simulink model "sk_Depositos_control"  (Simulink 8.9)
settings: Solver=ode45  StartTime=0.0  StopTime=tsim  RelTol=1e-3  EnableMultiTasking=on
values from neighbouring files (symbols this model uses):
  Tm = 10    [Proyecto.m]
settings Model: Creator=ortega  LastModifiedBy=javi_  ExtModeTrigMode=oneshot  ExtModeArmWhenConnect=off
settings DataIOCC: LimitDataPoints=off
settings OptimizationCC: BlockReduction=off  BooleanDataType=off  ExpressionDepthLimit=2147483647  InitFltsAndDblsToZero=on
settings DebuggingCC: SaveWithParameterizedLinksMsg=none  SignalResolutionControl=TryResolveAllWithWarning  MultiTaskDSMMsg=warning  MultiTaskCondExecSysMsg=none
settings HardwareCC: TargetUnknown=on
settings GRTTargetCC: ModelReferenceCompliant=off  CompOptLevelCompliant=off  GeneratePreprocessorConditionals=Use local settings  MatFileLogging=off

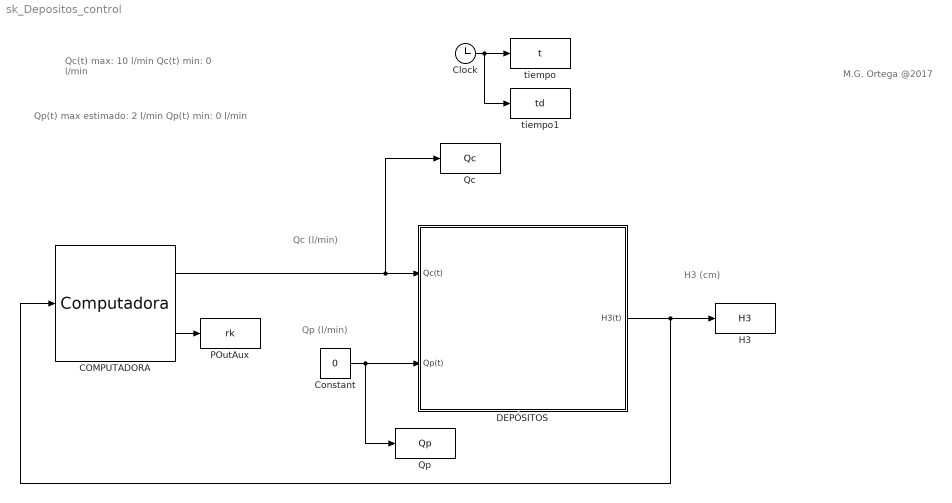
== system sk_Depositos_control ==
  note: Qc(t) max: 10 l/min
      | Qc(t) min:    0 l/min
  note: H3 (cm)
  note: Qc (l/min)
  note: Qp (l/min)
  note: Qp(t) max estimado: 2 l/min
      | Qp(t) min:    0 l/min
  note: M.G. Ortega @2017
  COMPUTADORA : S-Function  FunctionName=Computadora  Parameters=Tm  SFunctionDeploymentMode=off  EnableBusSupport=off  mask(Controlador){Tm=Tm}
      mask prompts: Tm "Tiempo de muestreo"
      mask help:
      | ENTRADAS:
      |   -  Salida del sistema: Yk
      |
      | SALIDAS:
      |   -  Señal de control: Ureal
      |   -  Puerto de salida auxiliar: POutAux
      mask Help:
      | Estos nombres no deberán ser modificados.
      | 
      |   El tiempo de muestreo se especifica mediante el único parámetro que se introduce desde Simulink
      |   En caso de ser utilizado en el código, su nombre será Tm.
      | 
      |   El alumno deberá modificar, en caso necesario, los siguiente ficheros:
      |   - Directivas.c
      |   - Declaraciones.c
      |   - Inicializaciones.c
      |   - Controlador.c
      | 
      | Autor: M.G. Ortega (2017)
      mask Display: image(imread('Computadora.jpg'))
  Clock : Clock
  Constant : Constant  Value=0
  DEPÓSITOS : Subsystem  mask{A1=40, A2=10, A3=30}
      mask prompts: A1 "Área del depósito 1 (cm^2)"; A2 "Área del depósito 2 (cm^2)"; A3 "Área del depósito 1 (cm^2)"
      mask help: SISTEMA CON TRES DEPÓSITOS EN SERIE
      mask Display: image(imread('Depositos.JPG'))
  H3 : ToWorkspace  VariableName=H3  SampleTime=-1
  POutAux : ToWorkspace  VariableName=rk
  Qc : ToWorkspace  VariableName=Qc
  Qp : ToWorkspace  VariableName=Qp  SampleTime=-1
  tiempo : ToWorkspace  VariableName=t  SampleTime=-1
  tiempo1 : ToWorkspace  VariableName=td  SampleTime=Tm
  wires:
  Constant/1 -> DEPÓSITOS/2(Qp(t)), Qp/1
  DEPÓSITOS/1(H3(t)) -> H3/1, COMPUTADORA/1
  Clock/1 -> tiempo1/1, tiempo/1
  COMPUTADORA/1 -> DEPÓSITOS/1(Qc(t)), Qc/1
  COMPUTADORA/2 -> POutAux/1

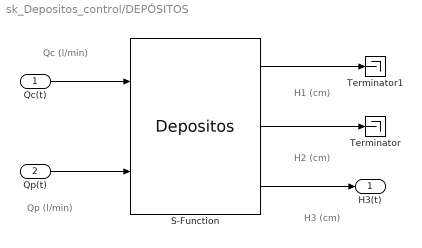
== system sk_Depositos_control/DEPÓSITOS ==
  note: H3 (cm)
  note: Qc (l/min)
  note: Qp (l/min)
  note: H2 (cm)
  note: H1 (cm)
  Qc(t) : Inport
  Qp(t) : Inport  Port=2
  S-Function : S-Function  FunctionName=Depositos  Parameters=A1;A2; A3  SFunctionDeploymentMode=off  EnableBusSupport=off
  Terminator : Terminator
  Terminator1 : Terminator
  H3(t) : Outport
  wires:
  Qc(t)/1 -> S-Function/1
  Qp(t)/1 -> S-Function/2
  S-Function/3 -> H3(t)/1
  S-Function/2 -> Terminator/1
  S-Function/1 -> Terminator1/1
